simulink model "PVHome"  (R2022b)
settings: Solver=FixedStepDiscrete  StartTime=0.0  StopTime=2  FixedStep=5e-6  RelTol=1e-3
undefined symbols (not defined in the file): Ion, Lithium
libraries: spsSeriesRLCBranchLib x175, spsBreakerLib x103, spsPWMGeneratorDCDCLib x94, spsThyristorLib x78, slpidlib x72, spsIGBTDiodeLib x62, spsThreePhaseVIMeasurementLib x59, spsThreePhaseBreakerLib x45, spsVoltageMeasurementLib x45, spsDiodeLib x39, spsThreePhaseParallelRLCBranchLib x38, spsMosfetLib x32
(part 16 of 16)

== matlab function PVHome/Subsystem6/MATLAB Function1 ==
  data: u input
function export_live_data(u)
% export_live_data  MATLAB Function block that writes 4 signals live into Excel
% Input: u (4-element vector)
% Exact workbook path used: 'V:\IEEE\LIVEdata.xlsx'
%
% Structure preserved: all COM/workspace actions run via evalin('base', ...)

    coder.extrinsic('evalin','assignin','actxserver','datetime','char','warning');

    persistent initialized
    if isempty(initialized)
        initialized = false;
    end

    % Convert inputs to doubles
    a = double(u(1)); b = double(u(2)); c = double(u(3)); d = double(u(4));

    % Use an .xlsx workbook for live UI updates
    excelPath = 'V:\IEEE\LIVEdata.csv';

    % Initialization block executed once (all logic runs inside evalin strings)
    if ~initialized
        % Ensure Excel COM server exists in base workspace and open/create workbook
        evalin('base', [ ...
            'if ~exist(''excelApp'',''var'') || isempty(excelApp), ' ...
                'excelApp = actxserver(''Excel.Application''); excelApp.Visible = true; ' ...
            'end; ' ...
            'if exist(''' excelPath ''',''file'')==2, ' ...
                'wb = excelApp.Workbooks.Open(''' excelPath '''); ws = wb.Worksheets.Item(1); ' ...
            'else, ' ...
                'wb = excelApp.Workbooks.Add; ws = wb.Worksheets.Item(1); ' ...
                'ws.Range(''A1'').Value = ''Timestamp''; ws.Range(''B1'').Value = ''Signal1''; ' ...
                'ws.Range(''C1'').Value = ''Signal2''; ws.Range(''D1'').Value = ''Signal3''; ' ...
                'ws.Range(''E1'').Value = ''Signal4''; wb.SaveAs(''' excelPath '''); ' ...
            'end; ' ...
            'if ~exist(''excelRow'',''var'') || isempty(excelRow), ur = ws.UsedRange; excelRow = double(ur.Rows.Count) + 1; end;']);

        initialized = true;
    end

    % Create timestamp string using datetime (host MATLAB)
    ts = char(datetime('now', 'Format', 'yyyy-MM-dd HH:mm:ss.SSS'));

    % Pass values into base workspace temporary variables (RHS only)
    assignin('base', 'tmp_ts', ts);
    assignin('base', 'tmp_a', a);
    assignin('base', 'tmp_b', b);
    assignin('base', 'tmp_c', c);
    assignin('base', 'tmp_d', d);

    % Perform the worksheet write and force Excel UI update (all inside evalin)
    % Note: r is the row written; we save, increment excelRow, then force repaint and scroll.
    evalin('base', [ ...
        'r = excelRow; ' ...
        'ws.Range([''A'' num2str(r)]).Value = tmp_ts; ' ...
        'ws.Range([''B'' num2str(r)]).Value = tmp_a; ' ...
        'ws.Range([''C'' num2str(r)]).Value = tmp_b; ' ...
        'ws.Range([''D'' num2str(r)]).Value = tmp_c; ' ...
        'ws.Range([''E'' num2str(r)]).Value = tmp_d; ' ...
        'wb.Save; ' ...
        'excelRow = r + 1; ' ...
        'try, excelApp.ScreenUpdating = true; excelApp.Calculate; ' ...
             'if ~isempty(excelApp.ActiveWindow), excelApp.ActiveWindow.ScrollRow = r; end; ' ...
             'pause(0.02); ' ...
        'end;']);

end

== matlab function PVHome/Subsystem4/Subsystem/MATLAB Function9 ==
  data: Sixty input; V_Consumer_Batter input; Wind_Breaker_Boost_Signal_Out output
function Wind_Breaker_Boost_Signal_Out = fcn(Sixty, V_Consumer_Batter)
Sixty = abs(Sixty);
V_Consumer_Batter = abs(V_Consumer_Batter);

D=1-(Sixty/V_Consumer_Batter);
Wind_Breaker_Boost_Signal_Out = D; %Vout

== matlab function PVHome/Subsystem3/Subsystem/MATLAB Function1 ==
  data: u input; y output
function y = fcn(u)
% This will output 1 - u
y = 1 - u;
